simulink model "simulink"  (R2022b)
settings: Solver=VariableStepAuto  StartTime=0.0  StopTime=1  RelTol=1e-3
values from neighbouring files (symbols this model uses):
  k = mean ( k_all )    [untitled.m]
  Tm = mean ( Tm_all )    [untitled.m]
  U = -100    [untitled.m]
settings Model: Creator=redmi  LastModifiedBy=Igor

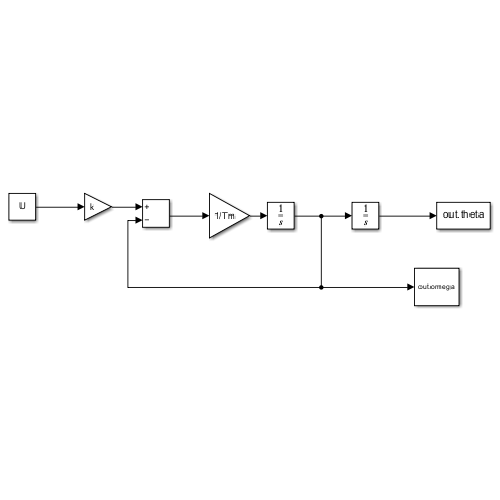
[thumbnail: Simulink's stored preview of the top-level diagram]
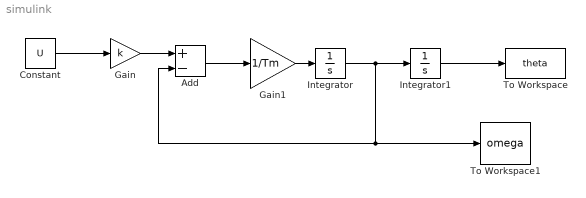
== system simulink ==
  Add : Sum  Inputs=+-
  Constant : Constant  Value=U
  Gain : Gain  Gain=k
  Gain1 : Gain  Gain=1/Tm
  Integrator : Integrator
  Integrator1 : Integrator
  To Workspace : ToWorkspace  VariableName=theta  SaveFormat=Timeseries  SampleTime=-1
  To Workspace1 : ToWorkspace  VariableName=omega  SaveFormat=Timeseries  SampleTime=-1
      settings: Save2DSignal=2-D array (concatenate along first dimension)
  wires:
  Constant/1 -> Gain/1
  Gain/1 -> Add/1
  Add/1 -> Gain1/1
  Gain1/1 -> Integrator/1
  Integrator/1 -> Integrator1/1, To Workspace1/1, Add/2
  Integrator1/1 -> To Workspace/1
